simulink model "diagrama3"  (R2022a)
settings: Solver=ode45  StartTime=0.0  StopTime=4.46  RelTol=1e-3  EnableMultiTasking=on
libraries: dspobslib x2, dspsigops x1, dspstat3 x1, dspsrcs4 x1
settings Model: Creator=tcom00  LastModifiedBy=oscar
settings SolverCC: AlgebraicLoopSolver=TrustRegion
settings DataIOCC: LimitDataPoints=on  SaveFormat=Array  SignalLoggingSaveFormat=ModelDataLogs  ReturnWorkspaceOutputs=off  SignalLoggingName=sigsOut
settings OptimizationCC: LifeSpan=inf
settings DebuggingCC: SaveWithParameterizedLinksMsg=none  UnderspecifiedInitializationDetection=Classic  MergeDetectMultiDrivingBlocksExec=none  SignalResolutionControl=TryResolveAllWithWarning  MultiTaskDSMMsg=warning  MultiTaskCondExecSysMsg=none  UnconnectedInputMsg=warning  UnconnectedOutputMsg=warning  UnconnectedLineMsg=warning  AllowSymbolicDim=off  SFUnexpectedBacktrackingDiag=warning  SFNoUnconditionalDefaultTransitionDiag=warning  SFExecutionAtInitializationDiag=none  SFMachineParentedDataDiag=warning  ArithmeticOperatorsInVariantConditions=warning
settings HardwareCC: ProdBitPerPointer=32  ProdBitPerSizeT=32  ProdBitPerPtrDiffT=32  ProdLargestAtomicFloat=None  ProdIntDivRoundTo=Undefined  ProdEndianess=Unspecified  ProdWordSize=32  ProdHWDeviceType=32-bit Generic  TargetUnknown=on
settings ModelReferenceCC: PropagateSignalLabelsOutOfModel=off
settings SFSimCC: SimUseLocalCustomCode=off  CustomCodeUndefinedFunction=UseInterfaceOnly
settings RTWCC: RTWUseLocalCustomCode=off
settings CodeAppCC: StateflowObjectComments=on
settings GRTTargetCC: TargetLangStandard=C89/C90 (ANSI)  CombineOutputUpdateFcns=off  GRTInterface=on
settings ConfigComp: CovMetricSettings=dw  CovSaveCumulativeToWorkspaceVar=on  CovSaveSingleToWorkspaceVar=on  CovExternalEMLEnable=off

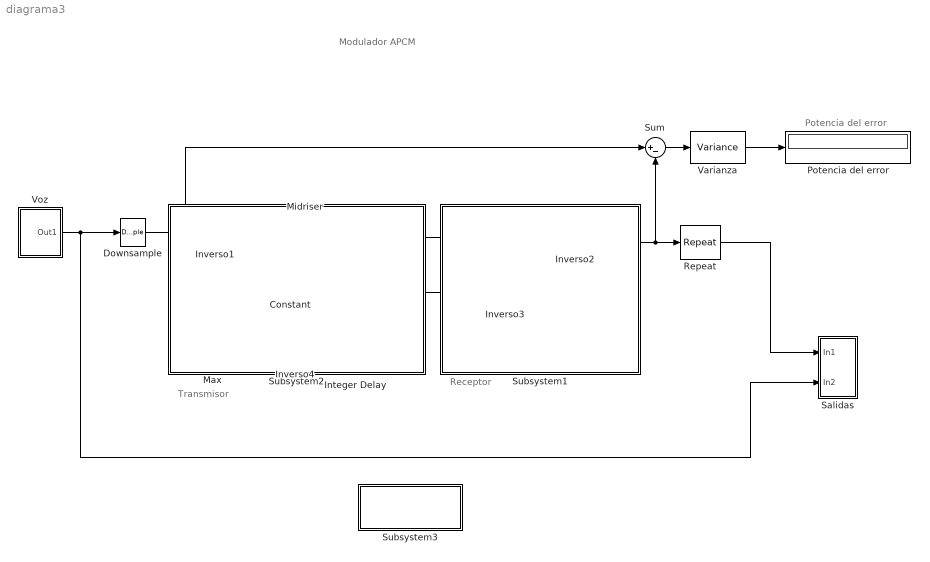
== system diagrama3 ==
  note: Transmisor
  note: Receptor
  note: Modulador APCM
  note: Potencia del error
  Constant : Constant
  Downsample : DownSample  N=4  InputProcessing=Inherited (this choice will be removed - see release notes)  RateOptions=Allow multirate processing
  Integer Delay : dspobslib/Integer Delay  delay=1  ic=1  reset_popup=None
      settings: SourceProductBaseCode=DS
  Inverso1 : Product  SaturateOnIntegerOverflow=on  OutDataTypeStr=Inherit: Same as first input
  Inverso2 : Product  SaturateOnIntegerOverflow=on  OutDataTypeStr=Inherit: Same as first input
  Inverso3 : Product  Inputs=/  SaturateOnIntegerOverflow=on  OutDataTypeStr=Inherit: Same as first input
  Inverso4 : Product  Inputs=/  SaturateOnIntegerOverflow=on  OutDataTypeStr=Inherit: Same as first input
  Max : MinMax  Function=max  Inputs=2  InputSameDT=on  SaturateOnIntegerOverflow=on
  Midriser : Subsystem  mask{L=256, xsc=1}
      mask prompts: L "niveles"
      mask Display: image('.\png\midriser.png');
  Potencia del error : Display
  Repeat : dspsigops/Repeat  N=4  InputProcessing=Columns as channels (frame based)  RateOptions=Allow multirate processing  ic=0  mode=Unused parameter value
  Salidas : Subsystem
      mask Display:
      | plot([0, 1], [1, 1]);
      | plot([0, 0], [1, 0.5]);
      | plot([0, 1], [0.5, 0.5]);
      | plot([1, 1], [1, 0.5]);
      | disp('\n\nMulti\nscope');
  Subsystem1 : Subsystem
      mask Display: disp('');
  Subsystem2 : Subsystem
      mask Display: disp('');
  Subsystem3 : Subsystem  mask{L=256, xsc=1}
      mask prompts: L "Niveles :"; xsc "xsc :"
      mask Callback L:
      | L = get_param(gcb, 'L');
      | set_param([bdroot '/Midriser'], 'L',L);
      mask Callback xsc:
      | xsc = get_param(gcb, 'xsc');
      | set_param([bdroot '/Midriser'], 'xsc',xsc);
      mask Display: disp('Parametros del\nsistema');
  Sum : Sum  Inputs=|+-  SaturateOnIntegerOverflow=on
  Varianza : dspstat3/Variance  run=on  InputProcessing=Columns as channels (frame based)  reset_popup=None  directionMode=Each column  dimension=1  roiEnable=off  roiType=Rectangles  roiPortion=Entire ROI  roiOutput=Individual statistics for each ROI  roiFlag=off  roundingMode=Floor  overflowMode=off
  Voz : Subsystem
      mask Display: disp('Voz');
  wires:
  Sum/1 -> Varianza/1
  Varianza/1 -> Potencia del error/1
  Downsample/1 -> Sum/1, Inverso1/1
  Midriser/1(Out1) -> Inverso2/1, Integer Delay/1
  Inverso1/1 -> Midriser/1(In1)
  Max/1 -> Inverso3/1, Inverso1/2
  Inverso2/1 -> Repeat/1, Sum/2
  Integer Delay/1 -> Inverso4/1
  Inverso3/1 -> Inverso2/2
  Voz/1(Out1) -> Salidas/2(In2), Downsample/1
  Constant/1 -> Max/1
  Inverso4/1 -> Max/2
  Repeat/1 -> Salidas/1(In1)

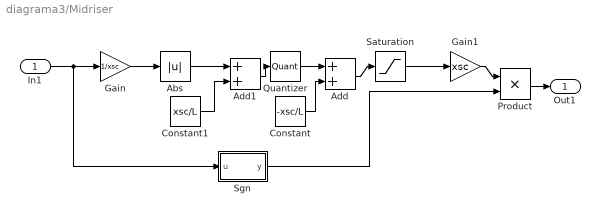
== system diagrama3/Midriser ==
  In1 : Inport
  Abs : Abs  SaturateOnIntegerOverflow=off
  Add : Sum
  Add1 : Sum
  Constant : Constant  Value=-xsc/L
  Constant1 : Constant  Value=xsc/L
  Gain : Gain  Gain=1/xsc
  Gain1 : Gain  Gain=xsc
  Product : Product
  Quantizer : Quantizer  QuantizationInterval=2*xsc/L
  Saturation : Saturate  UpperLimit=xsc-xsc/L  LowerLimit=-xsc+xsc/L
  Sgn : MATLAB Function  TreatAsAtomicUnit=on
  Out1 : Outport  VectorParamsAs1DForOutWhenUnconnected=off
  wires:
  In1/1 -> Gain/1, Sgn/1(u)
  Product/1 -> Out1/1
  Quantizer/1 -> Add/1
  Sgn/1(y) -> Product/2
  Constant/1 -> Add/2
  Add/1 -> Saturation/1
  Gain1/1 -> Product/1
  Saturation/1 -> Gain1/1
  Add1/1 -> Quantizer/1
  Gain/1 -> Abs/1
  Constant1/1 -> Add1/2
  Abs/1 -> Add1/1

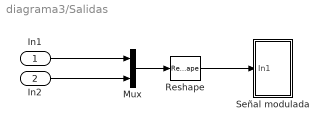
== system diagrama3/Salidas ==
  In1 : Inport
  In2 : Inport  Port=2
  Mux : Mux  Inputs=2
  Reshape : Reshape  OutputDimensionality=Row vector (2-D)
  Señal modulada : Subsystem
      mask Display:
      | plot([0, 1], [1, 1]);
      | plot([0, 0], [1, 0.5]);
      | plot([0, 1], [0.5, 0.5]);
      | plot([1, 1], [1, 0.5]);
      | disp('\n\nFrame\nscope');
  wires:
  Mux/1 -> Reshape/1
  Reshape/1 -> Señal modulada/1(In1)
  In1/1 -> Mux/1
  In2/1 -> Mux/2

== system diagrama3/Subsystem1 ==

== system diagrama3/Subsystem2 ==

== system diagrama3/Subsystem3 ==

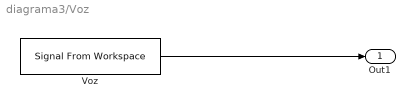
== system diagrama3/Voz ==
  Voz : dspsrcs4/Signal From Workspace  X=audioread('rtve1.wav')  Ts=1/8000  nsamps=1  OutputAfterFinalValue=Setting to zero  ignoreOrWarnInputAndFrameLengths=off  OutputFrames=on
  Out1 : Outport  VectorParamsAs1DForOutWhenUnconnected=off
  wires:
  Voz/1 -> Out1/1

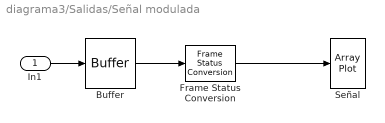
== system diagrama3/Salidas/Señal modulada ==
  In1 : Inport
  Buffer : Buffer  N=400
  Frame Status Conversion : dspobslib/Frame Status Conversion  growRefPort=off  outframe=Frame-based
      settings: SourceProductBaseCode=DS
  Señal : ArrayPlot  WindowPosition=[99.000000,439.000000,512.000000,300.000000,]  ScopeFrameLocation=window  PlotType=Line  AxesScaling=Manual  MaximizeAxes=Off  XLabel=Tiempo (s)  YLabel=Amplitud  YLimits=[-1.1,1.105]  ShowLegend=on  DefaultConfigurationName=dsp.scopes.ArrayPlotBlockSpecification
  wires:
  Buffer/1 -> Frame Status Conversion/1
  Frame Status Conversion/1 -> Señal/1
  In1/1 -> Buffer/1

== matlab function diagrama3/Midriser/Sgn ==
  data: u input; y output
function y = fcn(u)

if u~=0
    y=sign(u);
else
    y=1;
end
